simulink model "RefModel_SignalIntegrity"  (R2020a)
settings: Solver=ode1  StartTime=0.0  StopTime=10.0  FixedStep=Ts_SignalIntegrity.Ts_base  RelTol=1e-3
undefined symbols (not defined in the file or in its folder): ALGO_SET, IMU1, IMU2, IMU3, mag1, mag2, SIM_SENSOR_SET
(part 1 of 2)
settings Model: Creator=sl  LastModifiedBy=sl
settings OptimizationCC: DefaultParameterBehavior=Inlined  EnhancedBackFolding=on  PassReuseOutputArgsAs=Individual arguments  ZeroExternalMemoryAtStartup=off  ZeroInternalMemoryAtStartup=off  OptimizeBlockOrder=speed  DifferentSizesBufferReuse=on  OptimizationCustomize=off  EfficientTunableParamExpr=on
settings DebuggingCC: InheritedTsInSrcMsg=none  ParameterPrecisionLossMsg=none  ParameterTunabilityLossMsg=error  UnconnectedInputMsg=none  UnconnectedOutputMsg=none  UnconnectedLineMsg=none
settings HardwareCC: ProdBitPerPointer=32  ProdBitPerSizeT=32  ProdBitPerPtrDiffT=32  ProdLargestAtomicInteger=Long  ProdLargestAtomicFloat=Double  ProdWordSize=32  ProdHWDeviceType=ARM Compatible->ARM Cortex
settings ModelReferenceCC: ModelReferenceNumInstancesAllowed=Single
settings SFSimCC: MATLABDynamicMemAlloc=off
settings RTWCC: SystemTargetFile=ert.tlc  TemplateMakefile=ert_default_tmf  GenerateReport=on  IncludeHyperlinkInReport=on  LaunchReport=on  GenerateTraceInfo=on  GenerateTraceReport=on  GenerateTraceReportSl=on  GenerateTraceReportSf=on  GenerateTraceReportEml=on
settings CodeAppCC: ForceParamTrailComments=on  IgnoreCustomStorageClasses=off  MaxIdLength=48  OperatorAnnotations=on  SimulinkDataObjDesc=on  SFDataObjDesc=on  InsertBlockDesc=on
settings ERTTargetCC: TargetLangStandard=C99 (ISO)  GenerateSampleERTMain=on  LogVarNameModifier=none  SupportVariableSizeSignals=on  InlinedParameterPlacement=NonHierarchical  ERTCustomFileTemplate=example_file_process.tlc

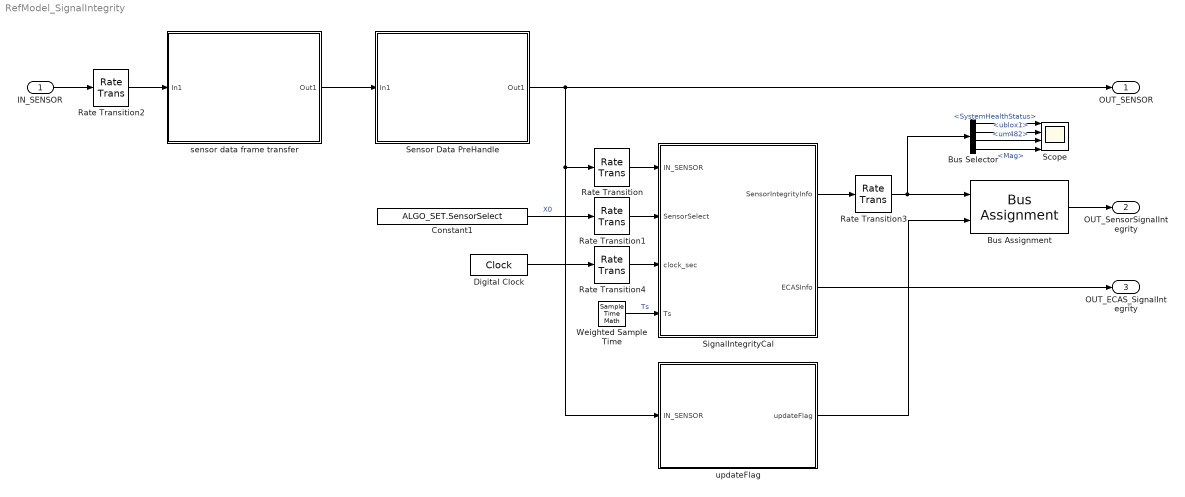
== system RefModel_SignalIntegrity ==
  IN_SENSOR : Inport  OutDataTypeStr=Bus: BUS_SENSOR  BusOutputAsStruct=on
  Bus Assignment : BusAssignment  AssignedSignals=SensorUpdateFlag
  Bus Selector : BusSelector  OutputSignals=SystemHealthStatus,SensorStatus.ublox1,SensorStatus.um482,SensorSelect.Mag
  Constant1 : Constant  Value=ALGO_SET.SensorSelect  OutDataTypeStr=Bus: BUS_NAVI_SensorSignalIntegrity_SensorSelect
  Digital Clock : DigitalClock  SampleTime=-1
  Rate Transition : RateTransition  Deterministic=off  OutPortSampleTime=Ts_SignalIntegrity.Ts_integrityCheck
  Rate Transition1 : RateTransition  Deterministic=off  OutPortSampleTime=Ts_SignalIntegrity.Ts_integrityCheck
  Rate Transition2 : RateTransition  Deterministic=off  OutPortSampleTime=Ts_SignalIntegrity.Ts_base
  Rate Transition3 : RateTransition  Deterministic=off
  Rate Transition4 : RateTransition  Deterministic=off  OutPortSampleTime=Ts_SignalIntegrity.Ts_integrityCheck
  Scope : Scope  NumInputPorts=4
  Sensor Data PreHandle : Subsystem
  SignalIntegrityCal : Stateflow chart  TreatAsAtomicUnit=on
  Weighted Sample Time : SampleTimeMath  TsampMathOp=Ts Only
  sensor data frame transfer : Subsystem
  updateFlag : Stateflow chart  TreatAsAtomicUnit=on
  OUT_SENSOR : Outport  OutDataTypeStr=Bus: BUS_SENSOR  BusOutputAsStruct=on
  OUT_SensorSignalIntegrity : Outport  Port=2  OutDataTypeStr=Bus: BUS_NAVI_SensorSignalIntegrity  BusOutputAsStruct=on
  OUT_ECAS_SignalIntegrity : Outport  Port=3  OutDataTypeStr=Bus: BUS_ECAS_SingalIntegrity  BusOutputAsStruct=on
  wires:
  Sensor Data PreHandle/1(Out1) -> Rate Transition/1, updateFlag/1(IN_SENSOR), OUT_SENSOR/1
  updateFlag/1(updateFlag) -> Bus Assignment/2
  Constant1/1 -> Rate Transition1/1  "X0"
  Digital Clock/1 -> Rate Transition4/1
  SignalIntegrityCal/1(SensorIntegrityInfo) -> Rate Transition3/1
  Rate Transition3/1 -> Bus Selector/1, Bus Assignment/1
  Rate Transition1/1 -> SignalIntegrityCal/2(SensorSelect)
  Rate Transition4/1 -> SignalIntegrityCal/3(clock_sec)
  Rate Transition/1 -> SignalIntegrityCal/1(IN_SENSOR)
  Rate Transition2/1 -> sensor data frame transfer/1(In1)
  Bus Assignment/1 -> OUT_SensorSignalIntegrity/1
  sensor data frame transfer/1(Out1) -> Sensor Data PreHandle/1(In1)
  IN_SENSOR/1 -> Rate Transition2/1
  Bus Selector/1 -> Scope/1  "<SystemHealthStatus>"
  Weighted Sample Time/1 -> SignalIntegrityCal/4(Ts)  "Ts"
  Bus Selector/2 -> Scope/2  "<ublox1>"
  Bus Selector/3 -> Scope/3  "<um482>"
  SignalIntegrityCal/2(ECASInfo) -> OUT_ECAS_SignalIntegrity/1
  Bus Selector/4 -> Scope/4  "<Mag>"

== system RefModel_SignalIntegrity/Sensor Data PreHandle ==
  In1 : Inport
  Manual Switch : ManualSwitch
  Sensor Data PreHandle : Subsystem  Commented=on
  Sensor Data PreHandle (No LowPass) : Subsystem
  Out1 : Outport
  wires:
  In1/1 -> Sensor Data PreHandle/1(In1), Sensor Data PreHandle (No LowPass)/1(In1)
  Sensor Data PreHandle/1(Out1) -> Manual Switch/2
  Sensor Data PreHandle (No LowPass)/1(Out1) -> Manual Switch/1
  Manual Switch/1 -> Out1/1

== system RefModel_SignalIntegrity/sensor data frame transfer ==
  In1 : Inport
  Bus Assignment : BusAssignment  AssignedSignals=IMU1,IMU2,IMU3,mag1,mag2
  Bus Selector : BusSelector  OutputSignals=IMU1,IMU2,IMU3
  Bus Selector1 : BusSelector  OutputSignals=mag1,mag2
  SensorFrame to BodyFrame : Subsystem
  SensorFrame to BodyFrame1 : Subsystem
  SensorFrame to BodyFrame2 : Subsystem
  SensorFrame to BodyFrame3 : Subsystem
  SensorFrame to BodyFrame4 : Subsystem
  Out1 : Outport
  wires:
  Bus Selector/1 -> SensorFrame to BodyFrame/1(In1)  "<IMU1>"
  Bus Selector/2 -> SensorFrame to BodyFrame1/1(In1)  "<IMU2>"
  Bus Selector/3 -> SensorFrame to BodyFrame2/1(In1)  "<IMU3>"
  SensorFrame to BodyFrame/1(Out1) -> Bus Assignment/2  "IMU1"
  SensorFrame to BodyFrame1/1(Out1) -> Bus Assignment/3  "IMU2"
  SensorFrame to BodyFrame2/1(Out1) -> Bus Assignment/4  "IMU3"
  Bus Assignment/1 -> Out1/1
  In1/1 -> Bus Selector1/1, Bus Assignment/1, Bus Selector/1
  Bus Selector1/1 -> SensorFrame to BodyFrame3/1(In1)  "<mag1>"
  Bus Selector1/2 -> SensorFrame to BodyFrame4/1(In1)  "<mag2>"
  SensorFrame to BodyFrame3/1(Out1) -> Bus Assignment/5  "mag1"
  SensorFrame to BodyFrame4/1(Out1) -> Bus Assignment/6  "mag2"

== system RefModel_SignalIntegrity/Sensor Data PreHandle/Sensor Data PreHandle ==
  In1 : Inport
  Bus Assignment : BusAssignment  AssignedSignals=IMU1,IMU2,IMU3,mag1,mag2
  Bus Selector : BusSelector  OutputSignals=IMU1,IMU2,IMU3
  Bus Selector1 : BusSelector  OutputSignals=mag1,mag2
  Subsystem : Subsystem
  Subsystem1 : Subsystem
  Subsystem2 : Subsystem
  Subsystem3 : Subsystem
  Subsystem4 : Subsystem
  Out1 : Outport
  wires:
  Subsystem/1(Out1) -> Bus Assignment/2  "IMU1"
  Subsystem1/1(Out1) -> Bus Assignment/3  "IMU2"
  Subsystem2/1(Out1) -> Bus Assignment/4  "IMU3"
  Bus Assignment/1 -> Out1/1
  In1/1 -> Bus Selector1/1, Bus Assignment/1, Bus Selector/1
  Subsystem3/1(Out1) -> Bus Assignment/5  "mag1"
  Subsystem4/1(Out1) -> Bus Assignment/6  "mag2"
  Bus Selector/1 -> Subsystem/1(In1)  "<IMU1>"
  Bus Selector/2 -> Subsystem1/1(In1)  "<IMU2>"
  Bus Selector/3 -> Subsystem2/1(In1)  "<IMU3>"
  Bus Selector1/1 -> Subsystem3/1(In1)  "<mag1>"
  Bus Selector1/2 -> Subsystem4/1(In1)  "<mag2>"

== system RefModel_SignalIntegrity/Sensor Data PreHandle/Sensor Data PreHandle (No LowPass) ==
  In1 : Inport
  Bus Assignment : BusAssignment  AssignedSignals=IMU1,IMU2,IMU3,mag1,mag2
  Bus Selector : BusSelector  OutputSignals=IMU1,IMU2,IMU3
  Bus Selector1 : BusSelector  OutputSignals=mag1,mag2
  Subsystem : Subsystem
  Subsystem1 : Subsystem
  Subsystem2 : Subsystem
  Subsystem3 : Subsystem
  Subsystem4 : Subsystem
  Out1 : Outport
  wires:
  Bus Selector1/2 -> Subsystem4/1(In1)  "<mag2>"
  Bus Selector1/1 -> Subsystem3/1(In1)  "<mag1>"
  Bus Selector/3 -> Subsystem2/1(In1)  "<IMU3>"
  Bus Selector/2 -> Subsystem1/1(In1)  "<IMU2>"
  Bus Selector/1 -> Subsystem/1(In1)  "<IMU1>"
  Subsystem4/1(Out1) -> Bus Assignment/6  "mag2"
  Subsystem3/1(Out1) -> Bus Assignment/5  "mag1"
  In1/1 -> Bus Selector/1, Bus Assignment/1, Bus Selector1/1
  Bus Assignment/1 -> Out1/1
  Subsystem2/1(Out1) -> Bus Assignment/4  "IMU3"
  Subsystem1/1(Out1) -> Bus Assignment/3  "IMU2"
  Subsystem/1(Out1) -> Bus Assignment/2  "IMU1"

== system RefModel_SignalIntegrity/sensor data frame transfer/SensorFrame to BodyFrame ==
  In1 : Inport
  Bus Creator : BusCreator  Inputs=7
  Bus Selector : BusSelector  OutputSignals=time,accel_x,accel_y,accel_z,gyro_x,gyro_y,gyro_z
  Frame Transfer : Subsystem
  Frame Transfer1 : Subsystem
  Out1 : Outport
  wires:
  Bus Selector/1 -> Bus Creator/1  "<time>"
  Bus Creator/1 -> Out1/1
  In1/1 -> Bus Selector/1
  Bus Selector/2 -> Frame Transfer/1(In1)  "<accel_x>"
  Bus Selector/3 -> Frame Transfer/2(In2)  "<accel_y>"
  Bus Selector/4 -> Frame Transfer/3(In3)  "<accel_z>"
  Frame Transfer/1(Out1) -> Bus Creator/2  "accel_x"
  Frame Transfer/2(Out2) -> Bus Creator/3  "accel_y"
  Frame Transfer/3(Out3) -> Bus Creator/4  "accel_z"
  Bus Selector/5 -> Frame Transfer1/1(In1)  "<gyro_x>"
  Bus Selector/6 -> Frame Transfer1/2(In2)  "<gyro_y>"
  Bus Selector/7 -> Frame Transfer1/3(In3)  "<gyro_z>"
  Frame Transfer1/1(Out1) -> Bus Creator/5  "gyro_x"
  Frame Transfer1/2(Out2) -> Bus Creator/6  "gyro_y"
  Frame Transfer1/3(Out3) -> Bus Creator/7  "gyro_z"

== system RefModel_SignalIntegrity/sensor data frame transfer/SensorFrame to BodyFrame1 ==
  In1 : Inport
  Bus Creator : BusCreator  Inputs=7
  Bus Selector : BusSelector  OutputSignals=time,accel_x,accel_y,accel_z,gyro_x,gyro_y,gyro_z
  Frame Transfer : Subsystem
  Frame Transfer1 : Subsystem
  Out1 : Outport
  wires:
  Frame Transfer1/3(Out3) -> Bus Creator/7  "gyro_z"
  Frame Transfer1/2(Out2) -> Bus Creator/6  "gyro_y"
  Frame Transfer1/1(Out1) -> Bus Creator/5  "gyro_x"
  Bus Selector/7 -> Frame Transfer1/3(In3)  "<gyro_z>"
  Bus Selector/6 -> Frame Transfer1/2(In2)  "<gyro_y>"
  Bus Selector/5 -> Frame Transfer1/1(In1)  "<gyro_x>"
  Frame Transfer/3(Out3) -> Bus Creator/4  "accel_z"
  Frame Transfer/2(Out2) -> Bus Creator/3  "accel_y"
  Frame Transfer/1(Out1) -> Bus Creator/2  "accel_x"
  Bus Selector/4 -> Frame Transfer/3(In3)  "<accel_z>"
  Bus Selector/3 -> Frame Transfer/2(In2)  "<accel_y>"
  Bus Selector/2 -> Frame Transfer/1(In1)  "<accel_x>"
  In1/1 -> Bus Selector/1
  Bus Creator/1 -> Out1/1
  Bus Selector/1 -> Bus Creator/1  "<time>"

== system RefModel_SignalIntegrity/sensor data frame transfer/SensorFrame to BodyFrame2 ==
  In1 : Inport
  Bus Creator : BusCreator  Inputs=7
  Bus Selector : BusSelector  OutputSignals=time,accel_x,accel_y,accel_z,gyro_x,gyro_y,gyro_z
  Frame Transfer : Subsystem
  Frame Transfer1 : Subsystem
  Out1 : Outport
  wires:
  Bus Selector/1 -> Bus Creator/1  "<time>"
  Bus Creator/1 -> Out1/1
  In1/1 -> Bus Selector/1
  Bus Selector/2 -> Frame Transfer/1(In1)  "<accel_x>"
  Bus Selector/3 -> Frame Transfer/2(In2)  "<accel_y>"
  Bus Selector/4 -> Frame Transfer/3(In3)  "<accel_z>"
  Frame Transfer/1(Out1) -> Bus Creator/2  "accel_x"
  Frame Transfer/2(Out2) -> Bus Creator/3  "accel_y"
  Frame Transfer/3(Out3) -> Bus Creator/4  "accel_z"
  Bus Selector/5 -> Frame Transfer1/1(In1)  "<gyro_x>"
  Bus Selector/6 -> Frame Transfer1/2(In2)  "<gyro_y>"
  Bus Selector/7 -> Frame Transfer1/3(In3)  "<gyro_z>"
  Frame Transfer1/1(Out1) -> Bus Creator/5  "gyro_x"
  Frame Transfer1/2(Out2) -> Bus Creator/6  "gyro_y"
  Frame Transfer1/3(Out3) -> Bus Creator/7  "gyro_z"

== system RefModel_SignalIntegrity/sensor data frame transfer/SensorFrame to BodyFrame3 ==
  In1 : Inport
  Bus Creator : BusCreator  Inputs=4
  Bus Selector : BusSelector  OutputSignals=time,mag_x,mag_y,mag_z
  Frame Transfer : Subsystem
  Out1 : Outport
  wires:
  Frame Transfer/3(Out3) -> Bus Creator/4  "mag_z"
  Frame Transfer/2(Out2) -> Bus Creator/3  "mag_y"
  Frame Transfer/1(Out1) -> Bus Creator/2  "mag_x"
  Bus Selector/4 -> Frame Transfer/3(In3)  "<mag_z>"
  Bus Selector/3 -> Frame Transfer/2(In2)  "<mag_y>"
  Bus Selector/2 -> Frame Transfer/1(In1)  "<mag_x>"
  In1/1 -> Bus Selector/1
  Bus Creator/1 -> Out1/1
  Bus Selector/1 -> Bus Creator/1  "<time>"

== system RefModel_SignalIntegrity/sensor data frame transfer/SensorFrame to BodyFrame4 ==
  In1 : Inport
  Bus Creator : BusCreator  Inputs=4
  Bus Selector : BusSelector  OutputSignals=time,mag_x,mag_y,mag_z
  Frame Transfer : Subsystem
  Out1 : Outport
  wires:
  Bus Selector/1 -> Bus Creator/1  "<time>"
  Bus Creator/1 -> Out1/1
  In1/1 -> Bus Selector/1
  Bus Selector/2 -> Frame Transfer/1(In1)  "<mag_x>"
  Bus Selector/3 -> Frame Transfer/2(In2)  "<mag_y>"
  Bus Selector/4 -> Frame Transfer/3(In3)  "<mag_z>"
  Frame Transfer/1(Out1) -> Bus Creator/2  "mag_x"
  Frame Transfer/2(Out2) -> Bus Creator/3  "mag_y"
  Frame Transfer/3(Out3) -> Bus Creator/4  "mag_z"

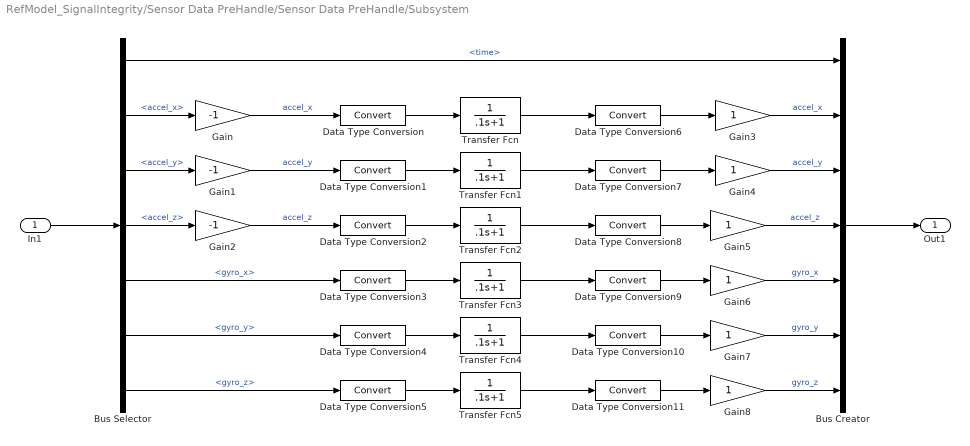
== system RefModel_SignalIntegrity/Sensor Data PreHandle/Sensor Data PreHandle/Subsystem ==
  In1 : Inport
  Bus Creator : BusCreator  Inputs=7
  Bus Selector : BusSelector  OutputSignals=time,accel_x,accel_y,accel_z,gyro_x,gyro_y,gyro_z
  Data Type Conversion{,1..11} (12 alike) : DataTypeConversion
  Gain : Gain  Gain=-1
  Gain1 : Gain  Gain=-1
  Gain2 : Gain  Gain=-1
  Gain{3..8} (6 alike) : Gain
  Transfer Fcn{,1..5} (6 alike) : TransferFcn  Denominator=[.1 1]
  Out1 : Outport
  wires:
  In1/1 -> Bus Selector/1
  Bus Creator/1 -> Out1/1
  Bus Selector/2 -> Gain/1  "<accel_x>"
  Bus Selector/3 -> Gain1/1  "<accel_y>"
  Bus Selector/4 -> Gain2/1  "<accel_z>"
  Bus Selector/1 -> Bus Creator/1  "<time>"
  Gain/1 -> Data Type Conversion/1  "accel_x"
  Gain1/1 -> Data Type Conversion1/1  "accel_y"
  Gain2/1 -> Data Type Conversion2/1  "accel_z"
  Bus Selector/5 -> Data Type Conversion3/1  "<gyro_x>"
  Bus Selector/6 -> Data Type Conversion4/1  "<gyro_y>"
  Bus Selector/7 -> Data Type Conversion5/1  "<gyro_z>"
  Gain3/1 -> Bus Creator/2  "accel_x"
  Gain4/1 -> Bus Creator/3  "accel_y"
  Gain5/1 -> Bus Creator/4  "accel_z"
  Gain6/1 -> Bus Creator/5  "gyro_x"
  Gain7/1 -> Bus Creator/6  "gyro_y"
  Gain8/1 -> Bus Creator/7  "gyro_z"
  Transfer Fcn/1 -> Data Type Conversion6/1
  Transfer Fcn1/1 -> Data Type Conversion7/1
  Transfer Fcn2/1 -> Data Type Conversion8/1
  Transfer Fcn3/1 -> Data Type Conversion9/1
  Transfer Fcn4/1 -> Data Type Conversion10/1
  Transfer Fcn5/1 -> Data Type Conversion11/1
  Data Type Conversion/1 -> Transfer Fcn/1
  Data Type Conversion1/1 -> Transfer Fcn1/1
  Data Type Conversion2/1 -> Transfer Fcn2/1
  Data Type Conversion5/1 -> Transfer Fcn5/1
  Data Type Conversion4/1 -> Transfer Fcn4/1
  Data Type Conversion3/1 -> Transfer Fcn3/1
  Data Type Conversion7/1 -> Gain4/1
  Data Type Conversion9/1 -> Gain6/1
  Data Type Conversion8/1 -> Gain5/1
  Data Type Conversion11/1 -> Gain8/1
  Data Type Conversion10/1 -> Gain7/1
  Data Type Conversion6/1 -> Gain3/1

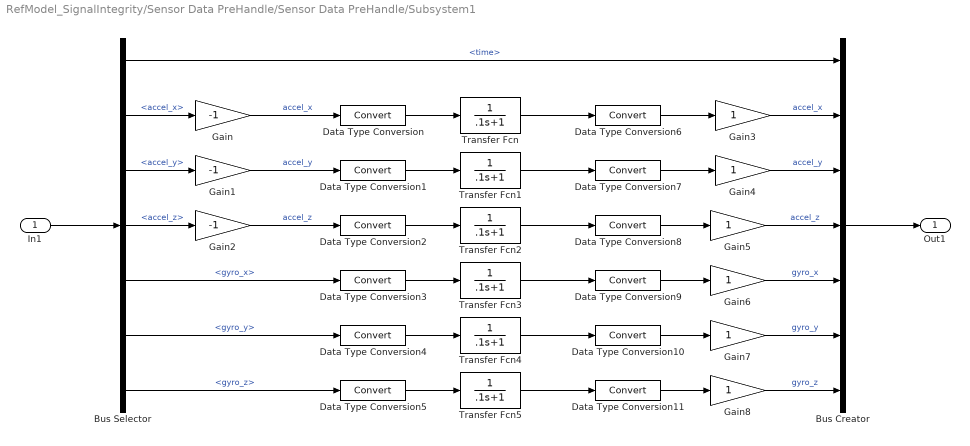
== system RefModel_SignalIntegrity/Sensor Data PreHandle/Sensor Data PreHandle/Subsystem1 ==
  In1 : Inport
  Bus Creator : BusCreator  Inputs=7
  Bus Selector : BusSelector  OutputSignals=time,accel_x,accel_y,accel_z,gyro_x,gyro_y,gyro_z
  Data Type Conversion{,1..11} (12 alike) : DataTypeConversion
  Gain : Gain  Gain=-1
  Gain1 : Gain  Gain=-1
  Gain2 : Gain  Gain=-1
  Gain{3..8} (6 alike) : Gain
  Transfer Fcn{,1..5} (6 alike) : TransferFcn  Denominator=[.1 1]
  Out1 : Outport
  wires:
  Data Type Conversion6/1 -> Gain3/1
  Data Type Conversion10/1 -> Gain7/1
  Data Type Conversion11/1 -> Gain8/1
  Data Type Conversion8/1 -> Gain5/1
  Data Type Conversion9/1 -> Gain6/1
  Data Type Conversion7/1 -> Gain4/1
  Data Type Conversion3/1 -> Transfer Fcn3/1
  Data Type Conversion4/1 -> Transfer Fcn4/1
  Data Type Conversion5/1 -> Transfer Fcn5/1
  Data Type Conversion2/1 -> Transfer Fcn2/1
  Data Type Conversion1/1 -> Transfer Fcn1/1
  Data Type Conversion/1 -> Transfer Fcn/1
  Transfer Fcn5/1 -> Data Type Conversion11/1
  Transfer Fcn4/1 -> Data Type Conversion10/1
  Transfer Fcn3/1 -> Data Type Conversion9/1
  Transfer Fcn2/1 -> Data Type Conversion8/1
  Transfer Fcn1/1 -> Data Type Conversion7/1
  Transfer Fcn/1 -> Data Type Conversion6/1
  Gain8/1 -> Bus Creator/7  "gyro_z"
  Gain7/1 -> Bus Creator/6  "gyro_y"
  Gain6/1 -> Bus Creator/5  "gyro_x"
  Gain5/1 -> Bus Creator/4  "accel_z"
  Gain4/1 -> Bus Creator/3  "accel_y"
  Gain3/1 -> Bus Creator/2  "accel_x"
  Bus Selector/7 -> Data Type Conversion5/1  "<gyro_z>"
  Bus Selector/6 -> Data Type Conversion4/1  "<gyro_y>"
  Bus Selector/5 -> Data Type Conversion3/1  "<gyro_x>"
  Gain2/1 -> Data Type Conversion2/1  "accel_z"
  Gain1/1 -> Data Type Conversion1/1  "accel_y"
  Gain/1 -> Data Type Conversion/1  "accel_x"
  Bus Selector/1 -> Bus Creator/1  "<time>"
  Bus Selector/4 -> Gain2/1  "<accel_z>"
  Bus Selector/3 -> Gain1/1  "<accel_y>"
  Bus Selector/2 -> Gain/1  "<accel_x>"
  Bus Creator/1 -> Out1/1
  In1/1 -> Bus Selector/1

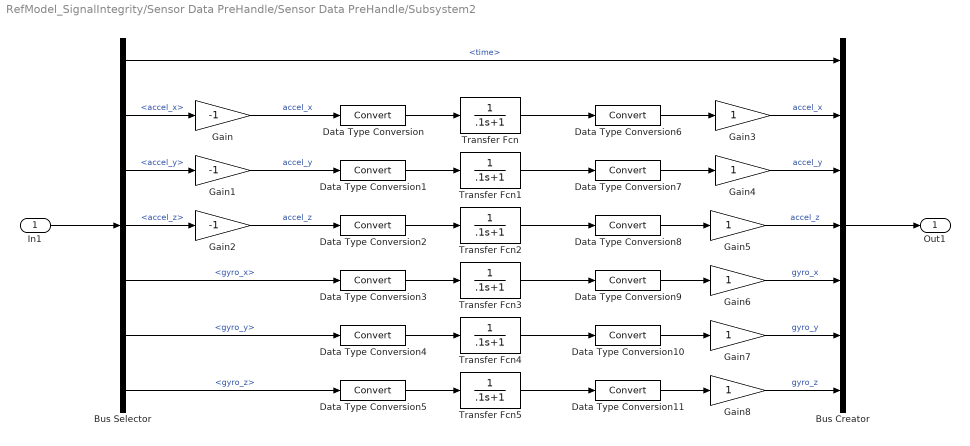
== system RefModel_SignalIntegrity/Sensor Data PreHandle/Sensor Data PreHandle/Subsystem2 ==
  In1 : Inport
  Bus Creator : BusCreator  Inputs=7
  Bus Selector : BusSelector  OutputSignals=time,accel_x,accel_y,accel_z,gyro_x,gyro_y,gyro_z
  Data Type Conversion{,1..11} (12 alike) : DataTypeConversion
  Gain : Gain  Gain=-1
  Gain1 : Gain  Gain=-1
  Gain2 : Gain  Gain=-1
  Gain{3..8} (6 alike) : Gain
  Transfer Fcn{,1..5} (6 alike) : TransferFcn  Denominator=[.1 1]
  Out1 : Outport
  wires:
  In1/1 -> Bus Selector/1
  Bus Creator/1 -> Out1/1
  Bus Selector/2 -> Gain/1  "<accel_x>"
  Bus Selector/3 -> Gain1/1  "<accel_y>"
  Bus Selector/4 -> Gain2/1  "<accel_z>"
  Bus Selector/1 -> Bus Creator/1  "<time>"
  Gain/1 -> Data Type Conversion/1  "accel_x"
  Gain1/1 -> Data Type Conversion1/1  "accel_y"
  Gain2/1 -> Data Type Conversion2/1  "accel_z"
  Bus Selector/5 -> Data Type Conversion3/1  "<gyro_x>"
  Bus Selector/6 -> Data Type Conversion4/1  "<gyro_y>"
  Bus Selector/7 -> Data Type Conversion5/1  "<gyro_z>"
  Gain3/1 -> Bus Creator/2  "accel_x"
  Gain4/1 -> Bus Creator/3  "accel_y"
  Gain5/1 -> Bus Creator/4  "accel_z"
  Gain6/1 -> Bus Creator/5  "gyro_x"
  Gain7/1 -> Bus Creator/6  "gyro_y"
  Gain8/1 -> Bus Creator/7  "gyro_z"
  Transfer Fcn/1 -> Data Type Conversion6/1
  Transfer Fcn1/1 -> Data Type Conversion7/1
  Transfer Fcn2/1 -> Data Type Conversion8/1
  Transfer Fcn3/1 -> Data Type Conversion9/1
  Transfer Fcn4/1 -> Data Type Conversion10/1
  Transfer Fcn5/1 -> Data Type Conversion11/1
  Data Type Conversion/1 -> Transfer Fcn/1
  Data Type Conversion1/1 -> Transfer Fcn1/1
  Data Type Conversion2/1 -> Transfer Fcn2/1
  Data Type Conversion5/1 -> Transfer Fcn5/1
  Data Type Conversion4/1 -> Transfer Fcn4/1
  Data Type Conversion3/1 -> Transfer Fcn3/1
  Data Type Conversion7/1 -> Gain4/1
  Data Type Conversion9/1 -> Gain6/1
  Data Type Conversion8/1 -> Gain5/1
  Data Type Conversion11/1 -> Gain8/1
  Data Type Conversion10/1 -> Gain7/1
  Data Type Conversion6/1 -> Gain3/1

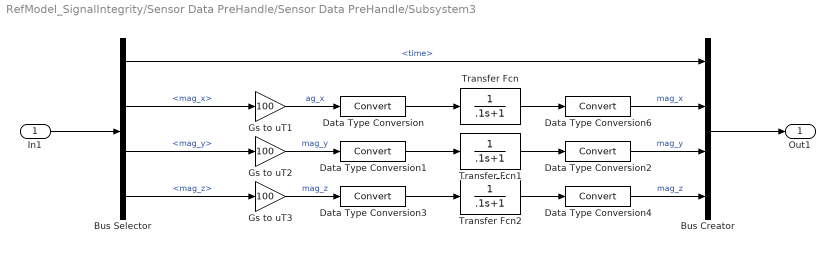
== system RefModel_SignalIntegrity/Sensor Data PreHandle/Sensor Data PreHandle/Subsystem3 ==
  In1 : Inport
  Bus Creator : BusCreator  Inputs=4
  Bus Selector : BusSelector  OutputSignals=time,mag_x,mag_y,mag_z
  Data Type Conversion{,1..4,6} (6 alike) : DataTypeConversion
  Gs to uT1 : Gain  Gain=100
  Gs to uT2 : Gain  Gain=100
  Gs to uT3 : Gain  Gain=100
  Transfer Fcn : TransferFcn  Denominator=[.1 1]
  Transfer Fcn1 : TransferFcn  Denominator=[.1 1]
  Transfer Fcn2 : TransferFcn  Denominator=[.1 1]
  Out1 : Outport
  wires:
  Bus Selector/1 -> Bus Creator/1  "<time>"
  Bus Creator/1 -> Out1/1
  In1/1 -> Bus Selector/1
  Bus Selector/2 -> Gs to uT1/1  "<mag_x>"
  Bus Selector/3 -> Gs to uT2/1  "<mag_y>"
  Bus Selector/4 -> Gs to uT3/1  "<mag_z>"
  Data Type Conversion/1 -> Transfer Fcn/1
  Transfer Fcn/1 -> Data Type Conversion6/1
  Data Type Conversion6/1 -> Bus Creator/2  "mag_x"
  Gs to uT1/1 -> Data Type Conversion/1  "ag_x"
  Transfer Fcn1/1 -> Data Type Conversion2/1
  Data Type Conversion1/1 -> Transfer Fcn1/1
  Data Type Conversion3/1 -> Transfer Fcn2/1
  Transfer Fcn2/1 -> Data Type Conversion4/1
  Gs to uT2/1 -> Data Type Conversion1/1  "mag_y"
  Gs to uT3/1 -> Data Type Conversion3/1  "mag_z"
  Data Type Conversion4/1 -> Bus Creator/4  "mag_z"
  Data Type Conversion2/1 -> Bus Creator/3  "mag_y"

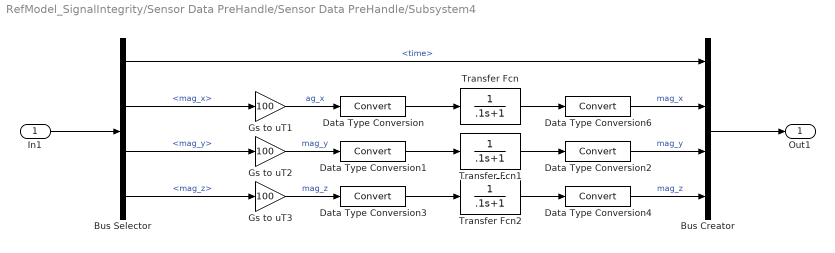
== system RefModel_SignalIntegrity/Sensor Data PreHandle/Sensor Data PreHandle/Subsystem4 ==
  In1 : Inport
  Bus Creator : BusCreator  Inputs=4
  Bus Selector : BusSelector  OutputSignals=time,mag_x,mag_y,mag_z
  Data Type Conversion{,1..4,6} (6 alike) : DataTypeConversion
  Gs to uT1 : Gain  Gain=100
  Gs to uT2 : Gain  Gain=100
  Gs to uT3 : Gain  Gain=100
  Transfer Fcn : TransferFcn  Denominator=[.1 1]
  Transfer Fcn1 : TransferFcn  Denominator=[.1 1]
  Transfer Fcn2 : TransferFcn  Denominator=[.1 1]
  Out1 : Outport
  wires:
  Data Type Conversion2/1 -> Bus Creator/3  "mag_y"
  Data Type Conversion4/1 -> Bus Creator/4  "mag_z"
  Gs to uT3/1 -> Data Type Conversion3/1  "mag_z"
  Gs to uT2/1 -> Data Type Conversion1/1  "mag_y"
  Transfer Fcn2/1 -> Data Type Conversion4/1
  Data Type Conversion3/1 -> Transfer Fcn2/1
  Data Type Conversion1/1 -> Transfer Fcn1/1
  Transfer Fcn1/1 -> Data Type Conversion2/1
  Gs to uT1/1 -> Data Type Conversion/1  "ag_x"
  Data Type Conversion6/1 -> Bus Creator/2  "mag_x"
  Transfer Fcn/1 -> Data Type Conversion6/1
  Data Type Conversion/1 -> Transfer Fcn/1
  Bus Selector/4 -> Gs to uT3/1  "<mag_z>"
  Bus Selector/3 -> Gs to uT2/1  "<mag_y>"
  Bus Selector/2 -> Gs to uT1/1  "<mag_x>"
  In1/1 -> Bus Selector/1
  Bus Creator/1 -> Out1/1
  Bus Selector/1 -> Bus Creator/1  "<time>"

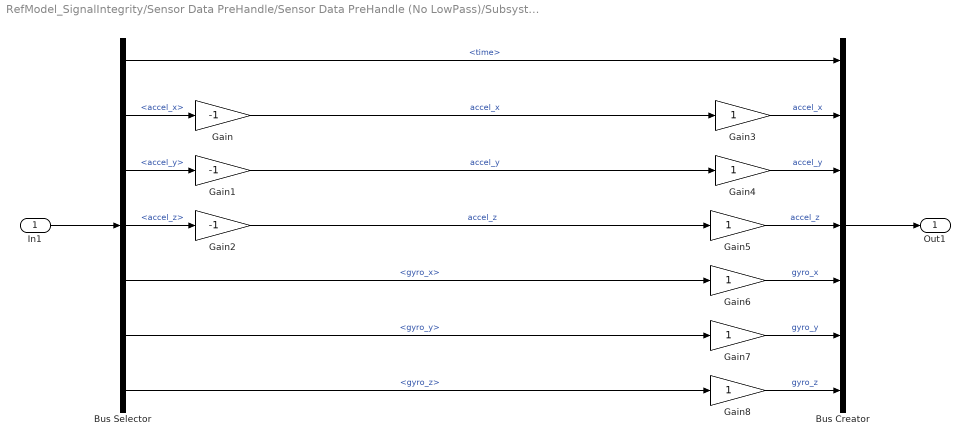
== system RefModel_SignalIntegrity/Sensor Data PreHandle/Sensor Data PreHandle (No LowPass)/Subsystem ==
  In1 : Inport
  Bus Creator : BusCreator  Inputs=7
  Bus Selector : BusSelector  OutputSignals=time,accel_x,accel_y,accel_z,gyro_x,gyro_y,gyro_z
  Gain : Gain  Gain=-1
  Gain1 : Gain  Gain=-1
  Gain2 : Gain  Gain=-1
  Gain{3..8} (6 alike) : Gain
  Out1 : Outport
  wires:
  Gain8/1 -> Bus Creator/7  "gyro_z"
  Gain7/1 -> Bus Creator/6  "gyro_y"
  Gain6/1 -> Bus Creator/5  "gyro_x"
  Gain5/1 -> Bus Creator/4  "accel_z"
  Gain4/1 -> Bus Creator/3  "accel_y"
  Gain3/1 -> Bus Creator/2  "accel_x"
  Bus Selector/7 -> Gain8/1  "<gyro_z>"
  Bus Selector/6 -> Gain7/1  "<gyro_y>"
  Bus Selector/5 -> Gain6/1  "<gyro_x>"
  Gain2/1 -> Gain5/1  "accel_z"
  Gain1/1 -> Gain4/1  "accel_y"
  Gain/1 -> Gain3/1  "accel_x"
  Bus Selector/1 -> Bus Creator/1  "<time>"
  Bus Selector/4 -> Gain2/1  "<accel_z>"
  Bus Selector/3 -> Gain1/1  "<accel_y>"
  Bus Selector/2 -> Gain/1  "<accel_x>"
  Bus Creator/1 -> Out1/1
  In1/1 -> Bus Selector/1

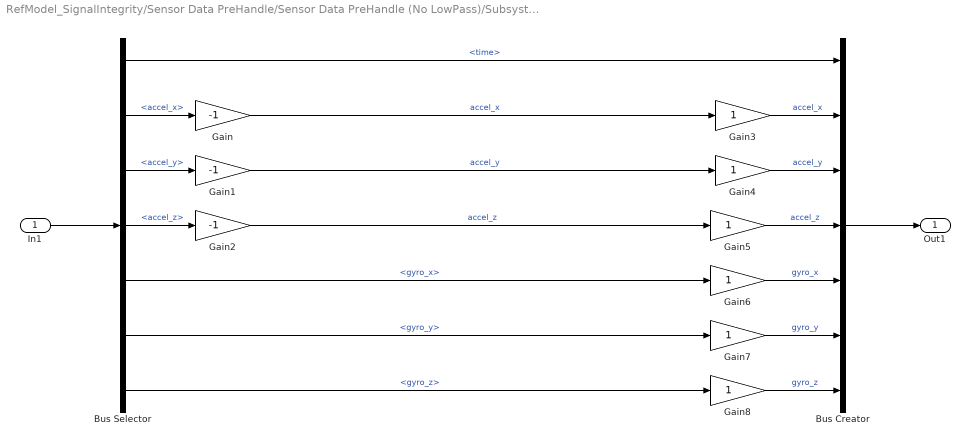
== system RefModel_SignalIntegrity/Sensor Data PreHandle/Sensor Data PreHandle (No LowPass)/Subsystem1 ==
  In1 : Inport
  Bus Creator : BusCreator  Inputs=7
  Bus Selector : BusSelector  OutputSignals=time,accel_x,accel_y,accel_z,gyro_x,gyro_y,gyro_z
  Gain : Gain  Gain=-1
  Gain1 : Gain  Gain=-1
  Gain2 : Gain  Gain=-1
  Gain{3..8} (6 alike) : Gain
  Out1 : Outport
  wires:
  In1/1 -> Bus Selector/1
  Bus Creator/1 -> Out1/1
  Bus Selector/2 -> Gain/1  "<accel_x>"
  Bus Selector/3 -> Gain1/1  "<accel_y>"
  Bus Selector/4 -> Gain2/1  "<accel_z>"
  Bus Selector/1 -> Bus Creator/1  "<time>"
  Gain/1 -> Gain3/1  "accel_x"
  Gain1/1 -> Gain4/1  "accel_y"
  Gain2/1 -> Gain5/1  "accel_z"
  Bus Selector/5 -> Gain6/1  "<gyro_x>"
  Bus Selector/6 -> Gain7/1  "<gyro_y>"
  Bus Selector/7 -> Gain8/1  "<gyro_z>"
  Gain3/1 -> Bus Creator/2  "accel_x"
  Gain4/1 -> Bus Creator/3  "accel_y"
  Gain5/1 -> Bus Creator/4  "accel_z"
  Gain6/1 -> Bus Creator/5  "gyro_x"
  Gain7/1 -> Bus Creator/6  "gyro_y"
  Gain8/1 -> Bus Creator/7  "gyro_z"

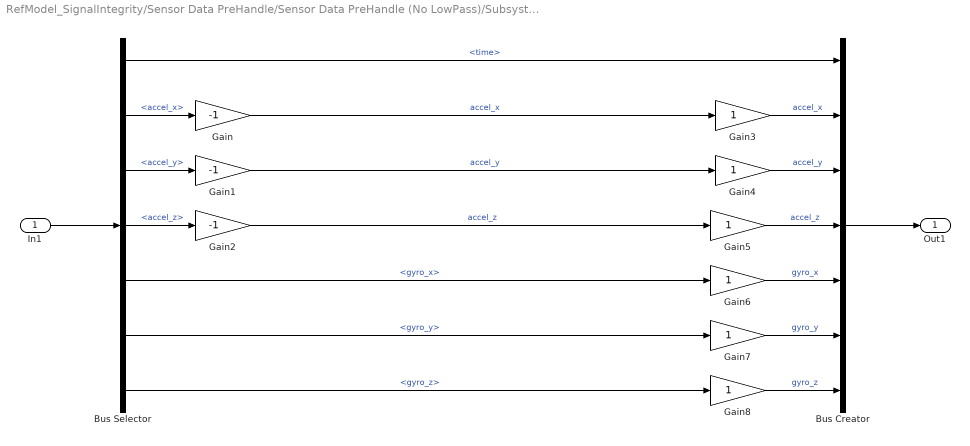
== system RefModel_SignalIntegrity/Sensor Data PreHandle/Sensor Data PreHandle (No LowPass)/Subsystem2 ==
  In1 : Inport
  Bus Creator : BusCreator  Inputs=7
  Bus Selector : BusSelector  OutputSignals=time,accel_x,accel_y,accel_z,gyro_x,gyro_y,gyro_z
  Gain : Gain  Gain=-1
  Gain1 : Gain  Gain=-1
  Gain2 : Gain  Gain=-1
  Gain{3..8} (6 alike) : Gain
  Out1 : Outport
  wires:
  Gain8/1 -> Bus Creator/7  "gyro_z"
  Gain7/1 -> Bus Creator/6  "gyro_y"
  Gain6/1 -> Bus Creator/5  "gyro_x"
  Gain5/1 -> Bus Creator/4  "accel_z"
  Gain4/1 -> Bus Creator/3  "accel_y"
  Gain3/1 -> Bus Creator/2  "accel_x"
  Bus Selector/7 -> Gain8/1  "<gyro_z>"
  Bus Selector/6 -> Gain7/1  "<gyro_y>"
  Bus Selector/5 -> Gain6/1  "<gyro_x>"
  Gain2/1 -> Gain5/1  "accel_z"
  Gain1/1 -> Gain4/1  "accel_y"
  Gain/1 -> Gain3/1  "accel_x"
  Bus Selector/1 -> Bus Creator/1  "<time>"
  Bus Selector/4 -> Gain2/1  "<accel_z>"
  Bus Selector/3 -> Gain1/1  "<accel_y>"
  Bus Selector/2 -> Gain/1  "<accel_x>"
  Bus Creator/1 -> Out1/1
  In1/1 -> Bus Selector/1

== system RefModel_SignalIntegrity/Sensor Data PreHandle/Sensor Data PreHandle (No LowPass)/Subsystem3 ==
  In1 : Inport
  Bus Creator : BusCreator  Inputs=4
  Bus Selector : BusSelector  OutputSignals=time,mag_x,mag_y,mag_z
  Gs to uT1 : Gain  Gain=100
  Gs to uT2 : Gain  Gain=100
  Gs to uT3 : Gain  Gain=100
  Out1 : Outport
  wires:
  Bus Selector/4 -> Gs to uT3/1  "<mag_z>"
  Bus Selector/3 -> Gs to uT2/1  "<mag_y>"
  Bus Selector/2 -> Gs to uT1/1  "<mag_x>"
  Gs to uT3/1 -> Bus Creator/4  "mag_z"
  Gs to uT2/1 -> Bus Creator/3  "mag_y"
  Gs to uT1/1 -> Bus Creator/2  "mag_x"
  In1/1 -> Bus Selector/1
  Bus Creator/1 -> Out1/1
  Bus Selector/1 -> Bus Creator/1  "<time>"

== system RefModel_SignalIntegrity/Sensor Data PreHandle/Sensor Data PreHandle (No LowPass)/Subsystem4 ==
  In1 : Inport
  Bus Creator : BusCreator  Inputs=4
  Bus Selector : BusSelector  OutputSignals=time,mag_x,mag_y,mag_z
  Gs to uT1 : Gain  Gain=100
  Gs to uT2 : Gain  Gain=100
  Gs to uT3 : Gain  Gain=100
  Out1 : Outport
  wires:
  Bus Selector/1 -> Bus Creator/1  "<time>"
  Bus Creator/1 -> Out1/1
  In1/1 -> Bus Selector/1
  Gs to uT1/1 -> Bus Creator/2  "mag_x"
  Gs to uT2/1 -> Bus Creator/3  "mag_y"
  Gs to uT3/1 -> Bus Creator/4  "mag_z"
  Bus Selector/2 -> Gs to uT1/1  "<mag_x>"
  Bus Selector/3 -> Gs to uT2/1  "<mag_y>"
  Bus Selector/4 -> Gs to uT3/1  "<mag_z>"

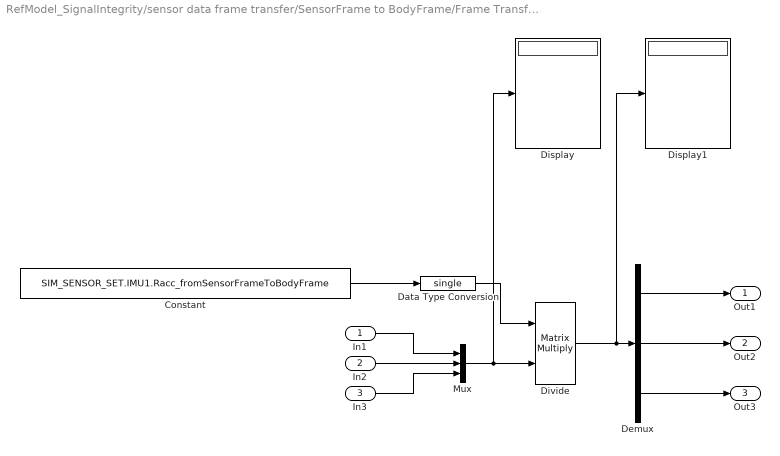
== system RefModel_SignalIntegrity/sensor data frame transfer/SensorFrame to BodyFrame/Frame Transfer ==
  In1 : Inport
  In2 : Inport  Port=2
  In3 : Inport  Port=3
  Constant : Constant  Value=SIM_SENSOR_SET.IMU1.Racc_fromSensorFrameToBodyFrame
  Data Type Conversion : DataTypeConversion  OutDataTypeStr=single
  Demux : Demux  Outputs=3
  Display : Display
  Display1 : Display
  Divide : Product  Inputs=**  Multiplication=Matrix(*)
  Mux : Mux  Inputs=3
  Out1 : Outport
  Out2 : Outport  Port=2
  Out3 : Outport  Port=3
  wires:
  In2/1 -> Mux/2
  In1/1 -> Mux/1
  In3/1 -> Mux/3
  Constant/1 -> Data Type Conversion/1
  Mux/1 -> Display/1, Divide/2
  Divide/1 -> Display1/1, Demux/1
  Demux/1 -> Out1/1
  Demux/2 -> Out2/1
  Demux/3 -> Out3/1
  Data Type Conversion/1 -> Divide/1

== system RefModel_SignalIntegrity/sensor data frame transfer/SensorFrame to BodyFrame/Frame Transfer1 ==
  In1 : Inport
  In2 : Inport  Port=2
  In3 : Inport  Port=3
  Constant : Constant  Value=SIM_SENSOR_SET.IMU1.Racc_fromSensorFrameToBodyFrame
  Data Type Conversion : DataTypeConversion  OutDataTypeStr=single
  Demux : Demux  Outputs=3
  Display : Display
  Display1 : Display
  Divide : Product  Inputs=**  Multiplication=Matrix(*)
  Mux : Mux  Inputs=3
  Out1 : Outport
  Out2 : Outport  Port=2
  Out3 : Outport  Port=3
  wires:
  Data Type Conversion/1 -> Divide/1
  Demux/3 -> Out3/1
  Demux/2 -> Out2/1
  Demux/1 -> Out1/1
  Divide/1 -> Demux/1, Display1/1
  Mux/1 -> Divide/2, Display/1
  Constant/1 -> Data Type Conversion/1
  In3/1 -> Mux/3
  In1/1 -> Mux/1
  In2/1 -> Mux/2

== system RefModel_SignalIntegrity/sensor data frame transfer/SensorFrame to BodyFrame1/Frame Transfer ==
  In1 : Inport
  In2 : Inport  Port=2
  In3 : Inport  Port=3
  Constant : Constant  Value=SIM_SENSOR_SET.IMU1.Racc_fromSensorFrameToBodyFrame
  Data Type Conversion : DataTypeConversion  OutDataTypeStr=single
  Demux : Demux  Outputs=3
  Display : Display
  Display1 : Display
  Divide : Product  Inputs=**  Multiplication=Matrix(*)
  Mux : Mux  Inputs=3
  Out1 : Outport
  Out2 : Outport  Port=2
  Out3 : Outport  Port=3
  wires:
  Data Type Conversion/1 -> Divide/1
  Demux/3 -> Out3/1
  Demux/2 -> Out2/1
  Demux/1 -> Out1/1
  Divide/1 -> Demux/1, Display1/1
  Mux/1 -> Divide/2, Display/1
  Constant/1 -> Data Type Conversion/1
  In3/1 -> Mux/3
  In1/1 -> Mux/1
  In2/1 -> Mux/2

== system RefModel_SignalIntegrity/sensor data frame transfer/SensorFrame to BodyFrame1/Frame Transfer1 ==
  In1 : Inport
  In2 : Inport  Port=2
  In3 : Inport  Port=3
  Constant : Constant  Value=SIM_SENSOR_SET.IMU1.Racc_fromSensorFrameToBodyFrame
  Data Type Conversion : DataTypeConversion  OutDataTypeStr=single
  Demux : Demux  Outputs=3
  Display : Display
  Display1 : Display
  Divide : Product  Inputs=**  Multiplication=Matrix(*)
  Mux : Mux  Inputs=3
  Out1 : Outport
  Out2 : Outport  Port=2
  Out3 : Outport  Port=3
  wires:
  In2/1 -> Mux/2
  In1/1 -> Mux/1
  In3/1 -> Mux/3
  Constant/1 -> Data Type Conversion/1
  Mux/1 -> Display/1, Divide/2
  Divide/1 -> Display1/1, Demux/1
  Demux/1 -> Out1/1
  Demux/2 -> Out2/1
  Demux/3 -> Out3/1
  Data Type Conversion/1 -> Divide/1

== system RefModel_SignalIntegrity/sensor data frame transfer/SensorFrame to BodyFrame2/Frame Transfer ==
  In1 : Inport
  In2 : Inport  Port=2
  In3 : Inport  Port=3
  Constant : Constant  Value=SIM_SENSOR_SET.IMU1.Racc_fromSensorFrameToBodyFrame
  Data Type Conversion : DataTypeConversion  OutDataTypeStr=single
  Demux : Demux  Outputs=3
  Display : Display
  Display1 : Display
  Divide : Product  Inputs=**  Multiplication=Matrix(*)
  Mux : Mux  Inputs=3
  Out1 : Outport
  Out2 : Outport  Port=2
  Out3 : Outport  Port=3
  wires:
  In2/1 -> Mux/2
  In1/1 -> Mux/1
  In3/1 -> Mux/3
  Constant/1 -> Data Type Conversion/1
  Mux/1 -> Display/1, Divide/2
  Divide/1 -> Display1/1, Demux/1
  Demux/1 -> Out1/1
  Demux/2 -> Out2/1
  Demux/3 -> Out3/1
  Data Type Conversion/1 -> Divide/1

== system RefModel_SignalIntegrity/sensor data frame transfer/SensorFrame to BodyFrame2/Frame Transfer1 ==
  In1 : Inport
  In2 : Inport  Port=2
  In3 : Inport  Port=3
  Constant : Constant  Value=SIM_SENSOR_SET.IMU1.Racc_fromSensorFrameToBodyFrame
  Data Type Conversion : DataTypeConversion  OutDataTypeStr=single
  Demux : Demux  Outputs=3
  Display : Display
  Display1 : Display
  Divide : Product  Inputs=**  Multiplication=Matrix(*)
  Mux : Mux  Inputs=3
  Out1 : Outport
  Out2 : Outport  Port=2
  Out3 : Outport  Port=3
  wires:
  Data Type Conversion/1 -> Divide/1
  Demux/3 -> Out3/1
  Demux/2 -> Out2/1
  Demux/1 -> Out1/1
  Divide/1 -> Demux/1, Display1/1
  Mux/1 -> Divide/2, Display/1
  Constant/1 -> Data Type Conversion/1
  In3/1 -> Mux/3
  In1/1 -> Mux/1
  In2/1 -> Mux/2

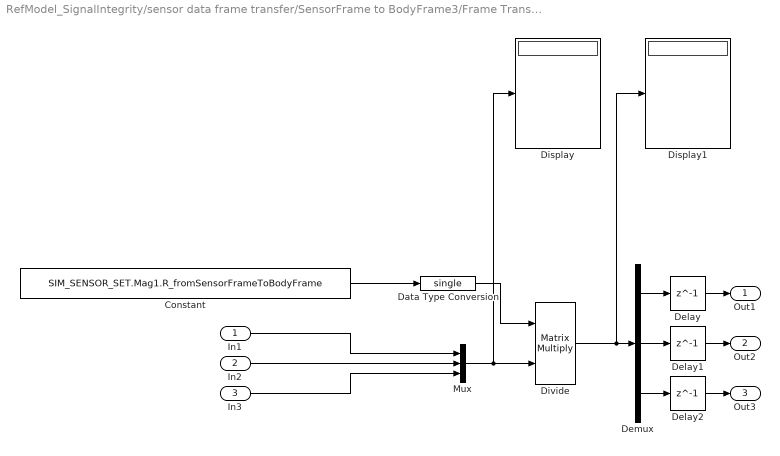
== system RefModel_SignalIntegrity/sensor data frame transfer/SensorFrame to BodyFrame3/Frame Transfer ==
  In1 : Inport
  In2 : Inport  Port=2
  In3 : Inport  Port=3
  Constant : Constant  Value=SIM_SENSOR_SET.Mag1.R_fromSensorFrameToBodyFrame
  Data Type Conversion : DataTypeConversion  OutDataTypeStr=single
  Delay : Delay  DelayLength=1
  Delay1 : Delay  DelayLength=1
  Delay2 : Delay  DelayLength=1
  Demux : Demux  Outputs=3
  Display : Display
  Display1 : Display
  Divide : Product  Inputs=**  Multiplication=Matrix(*)
  Mux : Mux  Inputs=3
  Out1 : Outport
  Out2 : Outport  Port=2
  Out3 : Outport  Port=3
  wires:
  Data Type Conversion/1 -> Divide/1
  Demux/3 -> Delay2/1
  Demux/2 -> Delay1/1
  Demux/1 -> Delay/1
  Divide/1 -> Demux/1, Display1/1
  Mux/1 -> Divide/2, Display/1
  Constant/1 -> Data Type Conversion/1
  In3/1 -> Mux/3
  In1/1 -> Mux/1
  In2/1 -> Mux/2
  Delay/1 -> Out1/1
  Delay1/1 -> Out2/1
  Delay2/1 -> Out3/1

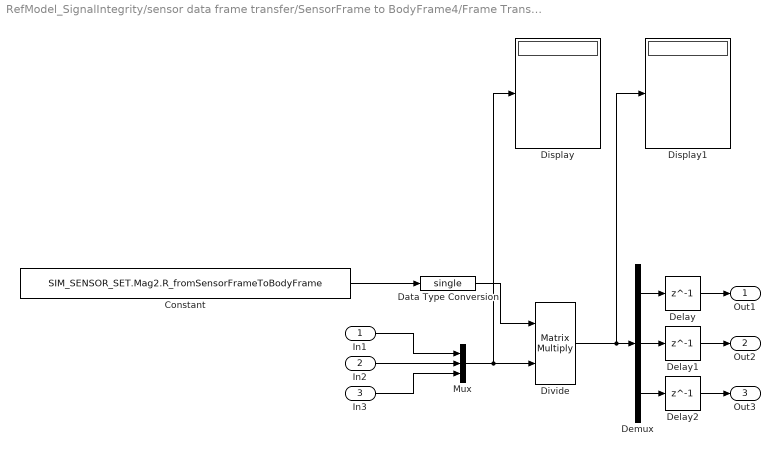
== system RefModel_SignalIntegrity/sensor data frame transfer/SensorFrame to BodyFrame4/Frame Transfer ==
  In1 : Inport
  In2 : Inport  Port=2
  In3 : Inport  Port=3
  Constant : Constant  Value=SIM_SENSOR_SET.Mag2.R_fromSensorFrameToBodyFrame
  Data Type Conversion : DataTypeConversion  OutDataTypeStr=single
  Delay : Delay  DelayLength=1
  Delay1 : Delay  DelayLength=1
  Delay2 : Delay  DelayLength=1
  Demux : Demux  Outputs=3
  Display : Display
  Display1 : Display
  Divide : Product  Inputs=**  Multiplication=Matrix(*)
  Mux : Mux  Inputs=3
  Out1 : Outport
  Out2 : Outport  Port=2
  Out3 : Outport  Port=3
  wires:
  In2/1 -> Mux/2
  In1/1 -> Mux/1
  In3/1 -> Mux/3
  Constant/1 -> Data Type Conversion/1
  Mux/1 -> Display/1, Divide/2
  Divide/1 -> Display1/1, Demux/1
  Demux/1 -> Delay/1
  Demux/2 -> Delay1/1
  Demux/3 -> Delay2/1
  Data Type Conversion/1 -> Divide/1
  Delay/1 -> Out1/1
  Delay2/1 -> Out3/1
  Delay1/1 -> Out2/1
